simulink subsystem "Med_PSM_Caudier"  (R2023a)
settings: Solver=VariableStepAuto  StartTime=0.0  StopTime=10.0  RelTol=1e-3
model mask{baseRobot=baseRobot, q0_=q0_}
  mask prompts: q0_ "q0_ (9 dim)"
settings Model: Creator=albher  LastModifiedBy=albher

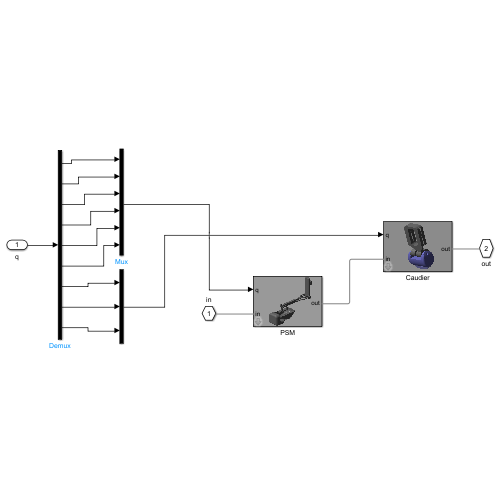
[thumbnail: Simulink's stored preview of the top-level diagram]
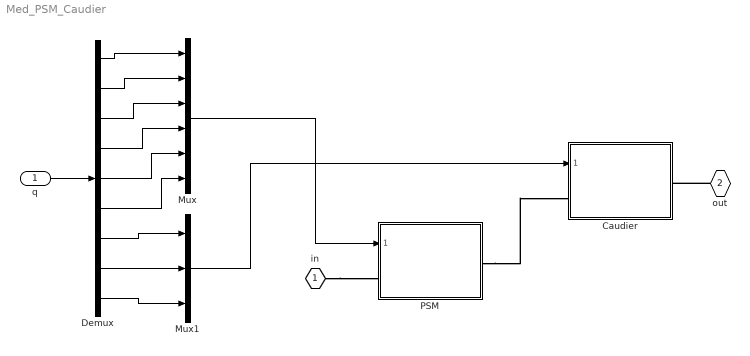
== system Med_PSM_Caudier ==
  q : Inport
  Caudier : Subsystem  ReferencedSubsystem=Med_Caudier  baseRobot=zeros(1:6)  q0_=q0_(7:9)
  Demux : Demux  Outputs=9
  Mux : Mux  Inputs=6
  Mux1 : Mux  Inputs=3
  PSM : Subsystem  ReferencedSubsystem=Med_PSM  baseRobot=baseRobot  q0_=q0_(1:6)
  in : PMIOPort  Side=Left
  out : PMIOPort  Port=2  Side=Right
  wires:
  q/1 -> Demux/1
  Demux/7 -> Mux1/1
  Demux/5 -> Mux/5
  Demux/3 -> Mux/3
  Demux/6 -> Mux/6
  Demux/8 -> Mux1/2
  Demux/2 -> Mux/2
  Demux/9 -> Mux1/3
  Demux/4 -> Mux/4
  Demux/1 -> Mux/1
  Mux/1 -> PSM/1
  Mux1/1 -> Caudier/1
  connections:
  in/RConn1 -- PSM/LConn1
  out/RConn1 -- Caudier/RConn1
  PSM/RConn1 -- Caudier/LConn1
